simulink model "ArmModelVersion2"  (R2013b)
settings: Solver=ode3  StartTime=0.0  StopTime=10.0  FixedStep=0.001  RelTol=1e-3
libraries: simulink x1
settings Model: Creator=Deepak  LastModifiedBy=Deepak
settings OptimizationCC: InlineParams=on

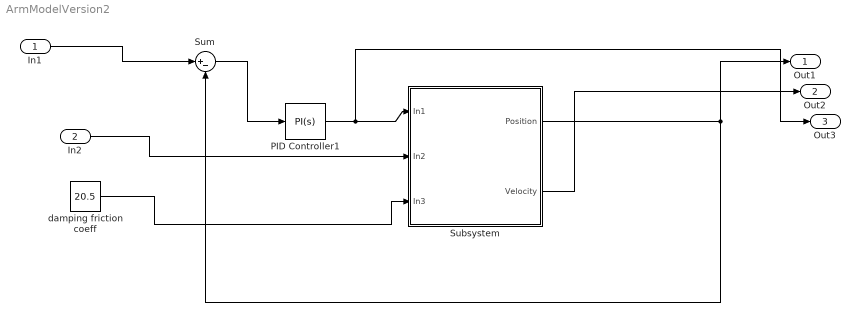
== system ArmModelVersion2 ==
  In1 : Inport
  In2 : Inport  Port=2
  PID Controller1 : simulink/Continuous/PID Controller  Controller=PI  TimeDomain=Continuous-time  SampleTime=-1  IntegratorMethod=Forward Euler  FilterMethod=Forward Euler  Form=Parallel  P=50000  I=1000.000721131539092422  D=1111.05906791895928  N=200.12291335792304  InitialConditionSource=internal  InitialConditionForIntegrator=0  InitialConditionForFilter=0  ExternalReset=none  LimitOutput=on  UpperSaturationLimit=200  LowerSaturationLimit=-200  LinearizeAsGain=on  AntiWindupMode=clamping  Kb=1  TrackingMode=off  Kt=1  PParamMin=[]  PParamMax=[]  IParamMin=[]  IParamMax=[]  DParamMin=[]  DParamMax=[]  NParamMin=[]  NParamMax=[]  KbParamMin=[]  KbParamMax=[]  KtParamMin=[]  KtParamMax=[]  POutMin=[]  POutMax=[]  IOutMin=[]  IOutMax=[]  DOutMin=[]  DOutMax=[]  NOutMin=[]  NOutMax=[]  KbOutMin=[]  KbOutMax=[]  KtOutMin=[]  KtOutMax=[]  IntegratorOutMin=[]  IntegratorOutMax=[]  FilterOutMin=[]  FilterOutMax=[]  SumOutMin=[]  SumOutMax=[]  SumI1OutMin=[]  SumI1OutMax=[]  SumI2OutMin=[]  SumI2OutMax=[]  SumI3OutMin=[]  SumI3OutMax=[]  SumDOutMin=[]  SumDOutMax=[]  SaturationOutMin=[]  SaturationOutMax=[]  IntegratorContinuousStateAttributes=''  IntegratorStateMustResolveToSignalObject=off  IntegratorRTWStateStorageClass=Auto  FilterContinuousStateAttributes=''  FilterStateMustResolveToSignalObject=off  FilterRTWStateStorageClass=Auto
      link override Filter: IntegratorMethod=Integration: Forward Euler  gainval=1.0  ExternalReset=none  InitialConditionSource=internal  InitialCondition=InitialConditionForFilter  InitialConditionMode=State only (most efficient)  SampleTime=-1  OutMin=FilterOutMin  OutMax=FilterOutMax  OutDataTypeStr=FilterOutDataTypeStr  LimitOutput=off  UpperSaturationLimit=inf  LowerSaturationLimit=-inf  ShowSaturationPort=off  ShowStatePort=off
      link override Filter: StateMustResolveToSignalObject=off
  Subsystem : Subsystem
  Sum : Sum  Inputs=|+-
  damping friction coeff : Constant  Value=20.5
  Out1 : Outport
  Out2 : Outport  Port=2
  Out3 : Outport  Port=3
  wires:
  Subsystem/1("Position ") -> Out1/1, Sum/2
  Subsystem/2(Velocity) -> Out2/1
  damping friction coeff/1 -> Subsystem/3(In3)
  Sum/1 -> PID Controller1/1
  PID Controller1/1 -> Out3/1, Subsystem/1(In1)
  In1/1 -> Sum/1
  In2/1 -> Subsystem/2(In2)

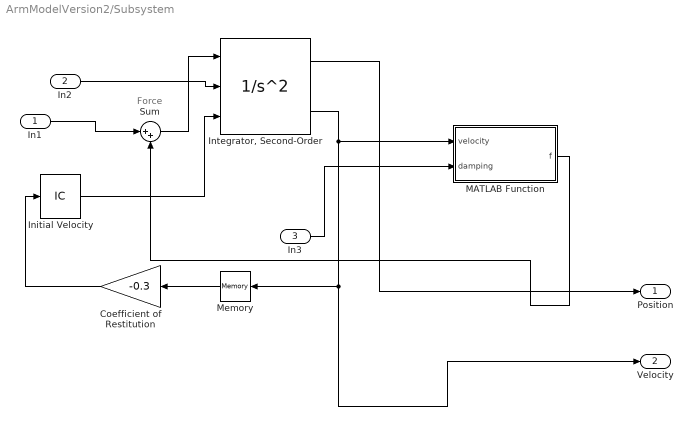
== system ArmModelVersion2/Subsystem ==
  note: Force
  In1 : Inport
  In2 : Inport  Port=2
  In3 : Inport  Port=3
  Coefficient of Restitution : Gain  Gain=-0.3
  "Initial Velocity " : InitialCondition  Value=0
  "Integrator, Second-Order" : SecondOrderIntegrator  ICSourceX=external  ICX=0.523  LimitX=on  LowerLimitX=-0.2623  ICSourceDXDT=external  ZeroCross=off  ReinitDXDTwhenXreachesSaturation=on
  MATLAB Function : MATLAB Function  TreatAsAtomicUnit=on
  Memory : Memory
  Sum : Sum  Inputs=|++
  "Position " : Outport
  Velocity : Outport  Port=2
  wires:
  In3/1 -> MATLAB Function/2(damping)
  "Integrator, Second-Order"/2 -> Memory/1, Velocity/1, MATLAB Function/1(velocity)
  MATLAB Function/1(f) -> Sum/2
  Sum/1 -> "Integrator, Second-Order"/1
  Memory/1 -> Coefficient of Restitution/1
  Coefficient of Restitution/1 -> "Initial Velocity "/1
  "Integrator, Second-Order"/1 -> "Position "/1
  In1/1 -> Sum/1
  "Initial Velocity "/1 -> "Integrator, Second-Order"/3
  In2/1 -> "Integrator, Second-Order"/2

== matlab function ArmModelVersion2/Subsystem/MATLAB Function ==
  data: velocity input; f output; damping input
function f = fcn(velocity, damping)
%#codegen

if abs(velocity) > 0.001
    f = -sign(velocity) * damping * abs(velocity) - 10.2; %A constant force always trying to decelerate the motion
else
    f = 0; % when the stick is not moving there are no net forces. 
end
